simulink model "lab3"  (R2016b)
settings: Solver=VariableStepAuto  StartTime=0.0  StopTime=250  RelTol=1e-3
settings Model: Creator=Admin  LastModifiedBy=Admin

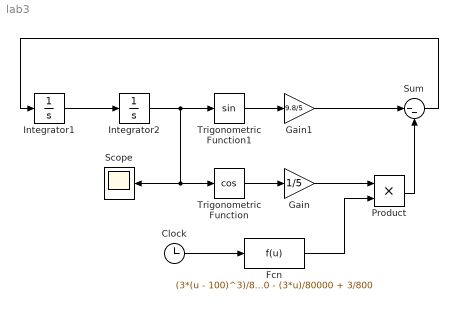
== system lab3 ==
  Clock : Clock
  Fcn : Fcn  Expr=(3*(u - 100)^3)/800000000 - (3*u)/80000 + 3/800
  Gain : Gain  Gain=1/5
  Gain1 : Gain  Gain=9.8/5
  Integrator1 : Integrator
  Integrator2 : Integrator
  Product : Product
  Scope : Scope
  Sum : Sum  Inputs=|--
  Trigonometric Function : Trigonometry  Operator=cos
  Trigonometric Function1 : Trigonometry
  wires:
  Sum/1 -> Integrator1/1
  Integrator1/1 -> Integrator2/1
  Integrator2/1 -> Trigonometric Function/1, Scope/1, Trigonometric Function1/1
  Trigonometric Function1/1 -> Gain1/1
  Gain1/1 -> Sum/1
  Product/1 -> Sum/2
  Gain/1 -> Product/1
  Trigonometric Function/1 -> Gain/1
  Clock/1 -> Fcn/1
  Fcn/1 -> Product/2
